simulink model "Copy_of_SeesawModelYeniRT_2015a"  (R2015a)
settings: Solver=ode3  StartTime=0.0  StopTime=Inf  FixedStep=0.01  RelTol=1e-3
values from neighbouring files (symbols this model uses):
  b = 1    [SeesawModel_parameters.m]
  g = 9.8    [SeesawModel_parameters.m]
  J = 1    [SeesawModel_parameters.m]
  K = 1    [SeesawModel_parameters.m]
  L = 1    [SeesawModel_parameters.m]
  md = 1    [SeesawModel_parameters.m]
  mp = 1    [SeesawModel_parameters.m]
  mr = 1    [SeesawModel_parameters.m]
  R = 1    [SeesawModel_parameters.m]
  rwheel = 1    [SeesawModel_parameters.m]
  testStep = 1    [SeesawModel_parameters.m]
  x1initial = 1    [SeesawModel_parameters.m]
  x2 = 1    [SeesawModel_parameters.m]
libraries: simulink x1, realtime_pacer_lib x1
settings Model: Creator=Administrator  LastModifiedBy=Administrator
settings SolverCC: EnableConcurrentExecution=on  ConcurrentTasks=on  AutoInsertRateTranBlk=on
settings DataIOCC: SaveFormat=StructureWithTime
settings OptimizationCC: BlockReduction=off  OptimizeBlockIOStorage=off  BufferReuse=off  GlobalBufferReuse=off  ExpressionFolding=off  LocalBlockOutputs=off
settings HardwareCC: ProdIntDivRoundTo=Zero  ProdEndianess=LittleEndian  ProdHWDeviceType=Generic->32-bit x86 compatible
settings RTWCC: SystemTargetFile=slrt.tlc  TemplateMakefile=slrt_default_tmf  Description=Simulink Real-Time  CodeExecutionProfiling=on  RTWCompilerOptimization=on
settings SimulinkRealTimeCC: SupportVariableSizeSignals=on  RL32LogTETModifier=off  xPCConcurrentTasks=on

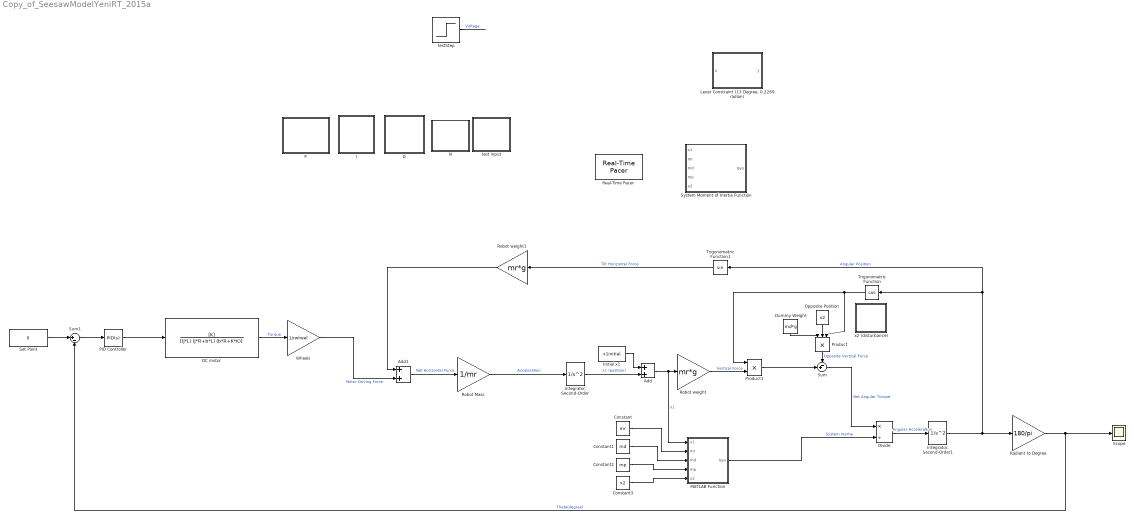
== system Copy_of_SeesawModelYeniRT_2015a ==
  Add : Sum
  Add1 : Sum
  Constant : Constant  Value=mr
  Constant1 : Constant  Value=md
  Constant2 : Constant  Value=mp
  Constant3 : Constant  Value=x2
  D : Subsystem  DialogController=hmiCreateDDGDialog  IsWebBlock=on  mask(MathWorksWebBlock){webBlockId=009f7443-6c34-401c-ab86-cf8c39a392cc, webBlockType=continuousknob, ShowInLibBrowser=on, ShowInitialText=on, HMISrcModelName=Copy_of_SeesawModelYeniRT_2015a}
      mask prompts: webBlockId "WebBlock Id"; webBlockType "WebBlock Type"; HMISrcModelName "Source Model"
      mask Help: helpview([docroot '/mapfiles/simulink.map'], 'hmi_knob')
      mask Display:
      | if strcmp(get_param(bdroot(gcb),'BlockDiagramType'), 'library')
      |     image([(matlabroot) '/toolbox/simulink/hmi/icons/ContinuousKnob.png']);
      | end
  DC motor : TransferFcn  Numerator=[K]  Denominator=[(J*L) (J*R+b*L) (b*R+K*K)]
  Divide : Product  Inputs=*/
  Dummy Weight : Constant  Value=md*g
  I : Subsystem  DialogController=hmiCreateDDGDialog  IsWebBlock=on  mask(MathWorksWebBlock){webBlockId=aeceef54-a51f-4b14-9b19-b68de4ed552d, webBlockType=continuousknob, ShowInLibBrowser=on, ShowInitialText=on, HMISrcModelName=Copy_of_SeesawModelYeniRT_2015a}
      mask prompts: webBlockId "WebBlock Id"; webBlockType "WebBlock Type"; HMISrcModelName "Source Model"
      mask Help: helpview([docroot '/mapfiles/simulink.map'], 'hmi_knob')
      mask Display:
      | if strcmp(get_param(bdroot(gcb),'BlockDiagramType'), 'library')
      |     image([(matlabroot) '/toolbox/simulink/hmi/icons/ContinuousKnob.png']);
      | end
  Initial x1 : Constant  Value=x1initial
  "Integrator, Second-Order" : SecondOrderIntegrator  LimitX=on  UpperLimitX=2  LowerLimitX=-2  ReinitDXDTwhenXreachesSaturation=on  ShowOutput=x
  "Integrator, Second-Order1" : SecondOrderIntegrator  ICX=0  LimitX=on  UpperLimitX=0.227  LowerLimitX=-0.227  ReinitDXDTwhenXreachesSaturation=on  ShowOutput=x
  "Lever Constraint (13 Degree, 0.2269 radian)" : MATLAB Function  TreatAsAtomicUnit=on
  MATLAB Function : MATLAB Function  TreatAsAtomicUnit=on
  N : Subsystem  DialogController=hmiCreateDDGDialog  IsWebBlock=on  mask(MathWorksWebBlock){webBlockId=232b09d2-61ff-42ce-84f6-fe5df92d27f0, webBlockType=continuousknob, ShowInLibBrowser=on, ShowInitialText=on, HMISrcModelName=Copy_of_SeesawModelYeniRT_2015a}
      mask prompts: webBlockId "WebBlock Id"; webBlockType "WebBlock Type"; HMISrcModelName "Source Model"
      mask Help: helpview([docroot '/mapfiles/simulink.map'], 'hmi_knob')
      mask Display:
      | if strcmp(get_param(bdroot(gcb),'BlockDiagramType'), 'library')
      |     image([(matlabroot) '/toolbox/simulink/hmi/icons/ContinuousKnob.png']);
      | end
  Opposite Position : Constant  Value=x2
  P : Subsystem  DialogController=hmiCreateDDGDialog  IsWebBlock=on  mask(MathWorksWebBlock){webBlockId=a6935ccc-1632-488c-b918-08dfa386d333, webBlockType=continuousknob, ShowInLibBrowser=on, ShowInitialText=on, HMISrcModelName=Copy_of_SeesawModelYeniRT_2015a}
      mask prompts: webBlockId "WebBlock Id"; webBlockType "WebBlock Type"; HMISrcModelName "Source Model"
      mask Help: helpview([docroot '/mapfiles/simulink.map'], 'hmi_knob')
      mask Display:
      | if strcmp(get_param(bdroot(gcb),'BlockDiagramType'), 'library')
      |     image([(matlabroot) '/toolbox/simulink/hmi/icons/ContinuousKnob.png']);
      | end
  PID Controller : simulink/Continuous/PID Controller  Controller=PID  TimeDomain=Continuous-time  SampleTime=-1  IntegratorMethod=Forward Euler  FilterMethod=Forward Euler  Form=Parallel  UseFilter=on  ControllerParametersSource=internal  P=0.2  I=4.8248  D=6.5525  N=184.4724  InitialConditionSource=internal  InitialConditionForIntegrator=0  InitialConditionForFilter=0  ExternalReset=none  LimitOutput=off  UpperSaturationLimit=inf  LowerSaturationLimit=-inf  LinearizeAsGain=on  AntiWindupMode=none  Kb=1  TrackingMode=off  Kt=1  PParamMin=[]  PParamMax=[]  IParamMin=[]  IParamMax=[]  DParamMin=[]  DParamMax=[]  NParamMin=[]  NParamMax=[]  KbParamMin=[]  KbParamMax=[]  KtParamMin=[]  KtParamMax=[]  POutMin=[]  POutMax=[]  IOutMin=[]  IOutMax=[]  DOutMin=[]  DOutMax=[]  NOutMin=[]  NOutMax=[]  KbOutMin=[]  KbOutMax=[]  KtOutMin=[]  KtOutMax=[]  IntegratorOutMin=[]  IntegratorOutMax=[]  FilterOutMin=[]  FilterOutMax=[]  SumOutMin=[]  SumOutMax=[]  SumI1OutMin=[]  SumI1OutMax=[]  SumI2OutMin=[]  SumI2OutMax=[]  SumI3OutMin=[]  SumI3OutMax=[]  SumDOutMin=[]  SumDOutMax=[]  SaturationOutMin=[]  SaturationOutMax=[]  IntegratorContinuousStateAttributes=''  IntegratorStateMustResolveToSignalObject=off  IntegratorRTWStateStorageClass=Auto  FilterContinuousStateAttributes=''  FilterStateMustResolveToSignalObject=off  FilterRTWStateStorageClass=Auto  DifferentiatorICPrevScaledInput=0  DifferentiatorOutMin=[]  DifferentiatorOutMax=[]
  Product : Product  Inputs=3
  Product1 : Product
  Radiant to Degree : Gain  Gain=180/pi
  Real-Time Pacer : realtime_pacer_lib/Real-Time Pacer  simTimePerRealTime=0.7
  Robot Mass : Gain  Gain=1/mr
  Robot weight : Gain  Gain=mr*g
  Robot weight1 : Gain  Gain=mr*g
  Scope : Scope
      settings: TimeRange=100  YMin=-15  YMax=15
  Set Point : Constant  Value=0
  Sum : Sum  Inputs=-+|
  Sum1 : Sum  Inputs=|+-
  System Moment of Inertia Function : MATLAB Function  TreatAsAtomicUnit=on
  Trigonometric Function : Trigonometry  Operator=cos
  Trigonometric Function1 : Trigonometry
  Wheels : Gain  Gain=1/rwheel
  test input : Subsystem  DialogController=hmiCreateDDGDialog  IsWebBlock=on  mask(MathWorksWebBlock){webBlockId=709484e7-e264-4911-b33e-5df9a1e1bddd, webBlockType=continuousknob, ShowInLibBrowser=on, ShowInitialText=on, HMISrcModelName=Copy_of_SeesawModelYeniRT_2015a}
      mask prompts: webBlockId "WebBlock Id"; webBlockType "WebBlock Type"; HMISrcModelName "Source Model"
      mask Help: helpview([docroot '/mapfiles/simulink.map'], 'hmi_knob')
      mask Display:
      | if strcmp(get_param(bdroot(gcb),'BlockDiagramType'), 'library')
      |     image([(matlabroot) '/toolbox/simulink/hmi/icons/ContinuousKnob.png']);
      | end
  testStep : Step  After=testStep  SampleTime=0
  x2 (disturbance) : Subsystem  DialogController=hmiCreateDDGDialog  IsWebBlock=on  mask(MathWorksWebBlock){webBlockId=b61cbe44-9a26-4ec6-8bd5-7c04f1a18c01, webBlockType=continuousknob, ShowInLibBrowser=on, ShowInitialText=on, HMISrcModelName=Copy_of_SeesawModelYeniRT_2015a}
      mask prompts: webBlockId "WebBlock Id"; webBlockType "WebBlock Type"; HMISrcModelName "Source Model"
      mask Help: helpview([docroot '/mapfiles/simulink.map'], 'hmi_knob')
      mask Display:
      | if strcmp(get_param(bdroot(gcb),'BlockDiagramType'), 'library')
      |     image([(matlabroot) '/toolbox/simulink/hmi/icons/ContinuousKnob.png']);
      | end
  wires:
  testStep/1 -> ?  "Voltage"
  DC motor/1 -> Wheels/1  "Torque"
  Wheels/1 -> Add1/2  "Motor Driving Force"
  Robot Mass/1 -> "Integrator, Second-Order"/1  "Acceleration"
  Dummy Weight/1 -> Product/1
  Opposite Position/1 -> Product/2
  Product/1 -> Sum/1  "Opposite Vertical Force"
  Robot weight/1 -> Product1/2  "Vertical Force"
  Sum/1 -> Divide/1  "Net Angular Torque"
  Divide/1 -> "Integrator, Second-Order1"/1  "Angular Acceleration"
  "Integrator, Second-Order1"/1 -> Radiant to Degree/1, Trigonometric Function/1, Trigonometric Function1/1  "Angular Position"
  MATLAB Function/1(Isys) -> Divide/2  "System Inertia"
  Constant/1 -> MATLAB Function/2(mr)
  Constant3/1 -> MATLAB Function/5(x2)
  Constant2/1 -> MATLAB Function/4(mp)
  Constant1/1 -> MATLAB Function/3(md)
  Radiant to Degree/1 -> Scope/1, Sum1/2  "Theta(degree)"
  Product1/1 -> Sum/2
  "Integrator, Second-Order"/1 -> Add/2  "x1 (position)"
  Add/1 -> MATLAB Function/1(x1), Robot weight/1  "x1"
  Initial x1/1 -> Add/1
  Trigonometric Function1/1 -> Robot weight1/1  "Tilt Horizontal Force"
  Add1/1 -> Robot Mass/1  "Net Horizontal Force"
  Trigonometric Function/1 -> Product/3, Product1/1
  Robot weight1/1 -> Add1/1
  PID Controller/1 -> DC motor/1
  Set Point/1 -> Sum1/1
  Sum1/1 -> PID Controller/1

== system Copy_of_SeesawModelYeniRT_2015a/D ==

== system Copy_of_SeesawModelYeniRT_2015a/I ==

== system Copy_of_SeesawModelYeniRT_2015a/N ==

== system Copy_of_SeesawModelYeniRT_2015a/P ==

== system Copy_of_SeesawModelYeniRT_2015a/test input ==

== system Copy_of_SeesawModelYeniRT_2015a/x2 (disturbance) ==

== matlab function Copy_of_SeesawModelYeniRT_2015a/Lever Constraint (13 Degree, 0.2269 radian) ==
  data: u input; y output
function y = leverConstraint(u)
if u>=0.2269    %0.2269=13*(pi/180)
    y=0.2269;
elseif u<=-0.2269
    y=-0.2269;
else
    y=u;
end

== matlab function Copy_of_SeesawModelYeniRT_2015a/System Moment of Inertia Function ==
  data: x1 input; Isys output; mr input; md input; mp input; x2 input
function Isys = Inertia(x1, mr, md, mp, x2)
M=mr+md+mp;
Mmasses=mr+md;
Isys=M*((Mmasses*((mr*x1+md*x2)/Mmasses))/M)^2;

== matlab function Copy_of_SeesawModelYeniRT_2015a/MATLAB Function ==
  data: x1 input; Isys output; mr input; md input; mp input; x2 input
function Isys = Inertia(x1, mr, md, mp, x2)
M=mr+md+mp;
Mmasses=mr+md;
CGm=(mr*x1-md*x2)/(mr+md);
CGs=(Mmasses*CGm)/M;
Isys=M*CGs^2;
